simulink model "LQRAirrefuelingYingHu_full"  (R2013a)
settings: Solver=ode45  StartTime=0.0  StopTime=100  RelTol=1e-3
values from neighbouring files (symbols this model uses):
  A_full = [A_full(1:7,1:7),zeros(7,1),A_full(1:7,8:11) ... (first row only)    [LQR_Calc2_F16YingHu_lonAndLa.m]
  B_full = [zeros(1,4);B(1:6,1:4);zeros(1,4);B(7:10,1:4)]    [LQR_Calc2_F16YingHu_lonAndLa.m]
  C_xd_h_yd = [C_xd_h,zeros(2,5) ... (first row only)    [LQR_Calc2_F16YingHu_lonAndLa.m]
  Ki = zeros(4,3)    [F16NolinearModelRemoveWindControlData_low.m]    (also in F16_2003hiModelAutopilot.m; F16_2003hiModelAutopilot1.m; LQR_Calc2.m = -k(:,9:10); LQR_Calc2LowPrecision.m = -k(:,9:10))
  Kp = zeros(4,18)    [F16NolinearModelRemoveWindControlData_low.m]    (also in F16_2003hiModelAutopilot.m; F16_2003hiModelAutopilot1.m; F16_2003hiModelAutopilot1_steadySys.m; LQR_Calc2.m = k(:,1:8))
libraries: simulink x3
settings Model: Creator=Dai  LastModifiedBy=Dai

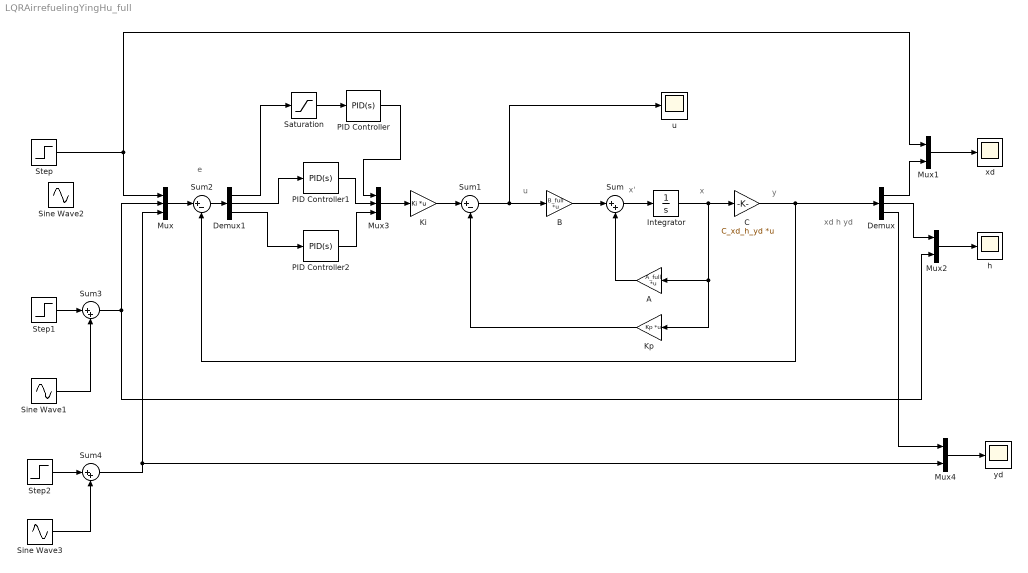
== system LQRAirrefuelingYingHu_full ==
  note: x
  note: x'
  note: y
  note: u
  note: xd
      | h
      | yd
  note: e
  A : Gain  Gain=A_full  Multiplication=Matrix(K*u) (u vector)
  B : Gain  Gain=B_full  Multiplication=Matrix(K*u) (u vector)
  C : Gain  Gain=C_xd_h_yd  Multiplication=Matrix(K*u) (u vector)
  Demux : Demux  Outputs=3
  Demux1 : Demux  Outputs=3
  Integrator : Integrator
  Ki : Gain  Gain=Ki  Multiplication=Matrix(K*u) (u vector)
  Kp : Gain  Gain=Kp  Multiplication=Matrix(K*u) (u vector)
  Mux : Mux  Inputs=3
  Mux1 : Mux  Inputs=2
  Mux2 : Mux  Inputs=2
  Mux3 : Mux  Inputs=3
  Mux4 : Mux  Inputs=2
  PID Controller : simulink/Continuous/PID Controller  Controller=PID  TimeDomain=Continuous-time  SampleTime=1  IntegratorMethod=Forward Euler  FilterMethod=Forward Euler  Form=Parallel  P=0  I=1.2  D=0  N=100  InitialConditionSource=internal  InitialConditionForIntegrator=0  InitialConditionForFilter=0  ExternalReset=none  LimitOutput=off  UpperSaturationLimit=inf  LowerSaturationLimit=-inf  LinearizeAsGain=on  AntiWindupMode=none  Kb=1  TrackingMode=off  Kt=1  PParamMin=[]  PParamMax=[]  IParamMin=[]  IParamMax=[]  DParamMin=[]  DParamMax=[]  NParamMin=[]  NParamMax=[]  KbParamMin=[]  KbParamMax=[]  KtParamMin=[]  KtParamMax=[]  POutMin=[]  POutMax=[]  IOutMin=[]  IOutMax=[]  DOutMin=[]  DOutMax=[]  NOutMin=[]  NOutMax=[]  KbOutMin=[]  KbOutMax=[]  KtOutMin=[]  KtOutMax=[]  IntegratorOutMin=[]  IntegratorOutMax=[]  FilterOutMin=[]  FilterOutMax=[]  SumOutMin=[]  SumOutMax=[]  SumI1OutMin=[]  SumI1OutMax=[]  SumI2OutMin=[]  SumI2OutMax=[]  SumI3OutMin=[]  SumI3OutMax=[]  SumDOutMin=[]  SumDOutMax=[]  SaturationOutMin=[]  SaturationOutMax=[]  IntegratorContinuousStateAttributes=''  IntegratorStateMustResolveToSignalObject=off  IntegratorRTWStateStorageClass=Auto  FilterContinuousStateAttributes=''  FilterStateMustResolveToSignalObject=off  FilterRTWStateStorageClass=Auto
  PID Controller1 : simulink/Continuous/PID Controller  Controller=PID  TimeDomain=Continuous-time  SampleTime=1  IntegratorMethod=Forward Euler  FilterMethod=Forward Euler  Form=Parallel  P=0  I=1.5  D=0  N=100  InitialConditionSource=internal  InitialConditionForIntegrator=0  InitialConditionForFilter=0  ExternalReset=none  LimitOutput=off  UpperSaturationLimit=inf  LowerSaturationLimit=-inf  LinearizeAsGain=on  AntiWindupMode=none  Kb=1  TrackingMode=off  Kt=1  PParamMin=[]  PParamMax=[]  IParamMin=[]  IParamMax=[]  DParamMin=[]  DParamMax=[]  NParamMin=[]  NParamMax=[]  KbParamMin=[]  KbParamMax=[]  KtParamMin=[]  KtParamMax=[]  POutMin=[]  POutMax=[]  IOutMin=[]  IOutMax=[]  DOutMin=[]  DOutMax=[]  NOutMin=[]  NOutMax=[]  KbOutMin=[]  KbOutMax=[]  KtOutMin=[]  KtOutMax=[]  IntegratorOutMin=[]  IntegratorOutMax=[]  FilterOutMin=[]  FilterOutMax=[]  SumOutMin=[]  SumOutMax=[]  SumI1OutMin=[]  SumI1OutMax=[]  SumI2OutMin=[]  SumI2OutMax=[]  SumI3OutMin=[]  SumI3OutMax=[]  SumDOutMin=[]  SumDOutMax=[]  SaturationOutMin=[]  SaturationOutMax=[]  IntegratorContinuousStateAttributes=''  IntegratorStateMustResolveToSignalObject=off  IntegratorRTWStateStorageClass=Auto  FilterContinuousStateAttributes=''  FilterStateMustResolveToSignalObject=off  FilterRTWStateStorageClass=Auto
  PID Controller2 : simulink/Continuous/PID Controller  Controller=PID  TimeDomain=Continuous-time  SampleTime=1  IntegratorMethod=Forward Euler  FilterMethod=Forward Euler  Form=Parallel  P=0  I=1  D=0  N=100  InitialConditionSource=internal  InitialConditionForIntegrator=0  InitialConditionForFilter=0  ExternalReset=none  LimitOutput=off  UpperSaturationLimit=inf  LowerSaturationLimit=-inf  LinearizeAsGain=on  AntiWindupMode=none  Kb=1  TrackingMode=off  Kt=1  PParamMin=[]  PParamMax=[]  IParamMin=[]  IParamMax=[]  DParamMin=[]  DParamMax=[]  NParamMin=[]  NParamMax=[]  KbParamMin=[]  KbParamMax=[]  KtParamMin=[]  KtParamMax=[]  POutMin=[]  POutMax=[]  IOutMin=[]  IOutMax=[]  DOutMin=[]  DOutMax=[]  NOutMin=[]  NOutMax=[]  KbOutMin=[]  KbOutMax=[]  KtOutMin=[]  KtOutMax=[]  IntegratorOutMin=[]  IntegratorOutMax=[]  FilterOutMin=[]  FilterOutMax=[]  SumOutMin=[]  SumOutMax=[]  SumI1OutMin=[]  SumI1OutMax=[]  SumI2OutMin=[]  SumI2OutMax=[]  SumI3OutMin=[]  SumI3OutMax=[]  SumDOutMin=[]  SumDOutMax=[]  SaturationOutMin=[]  SaturationOutMax=[]  IntegratorContinuousStateAttributes=''  IntegratorStateMustResolveToSignalObject=off  IntegratorRTWStateStorageClass=Auto  FilterContinuousStateAttributes=''  FilterStateMustResolveToSignalObject=off  FilterRTWStateStorageClass=Auto
  Saturation : Saturate
  Sine Wave1 : Sin  Amplitude=0.2  Frequency=0.05  SampleTime=0
  Sine Wave2 : Sin  Amplitude=5  Frequency=0.05  SampleTime=0
  Sine Wave3 : Sin  Amplitude=0.2  Frequency=0.05  SampleTime=0
  Step : Step  After=5  SampleTime=0
  Step1 : Step  Time=0  After=5  SampleTime=0
  Step2 : Step  Time=0  After=5  SampleTime=0
  Sum : Sum  Inputs=|++
  Sum1 : Sum  Inputs=|+-
  Sum2 : Sum  Inputs=|+-
  Sum3 : Sum  Inputs=|++
  Sum4 : Sum  Inputs=|++
  h : Scope
  u : Scope
      settings: SaveName=ScopeData2
  xd : Scope
  yd : Scope
      settings: SaveName=ScopeData3
  wires:
  Integrator/1 -> C/1, A/1, Kp/1
  B/1 -> Sum/1
  Sum/1 -> Integrator/1
  A/1 -> Sum/2
  Ki/1 -> Sum1/1
  C/1 -> Demux/1, Sum2/2
  Mux/1 -> Sum2/1
  Step/1 -> Mux/1, Mux1/1
  Demux/1 -> Mux1/2
  Mux1/1 -> xd/1
  Sum3/1 -> Mux2/2, Mux/2
  Mux2/1 -> h/1
  Demux/2 -> Mux2/1
  Kp/1 -> Sum1/2
  Sum2/1 -> Demux1/1
  Mux3/1 -> Ki/1
  Sum1/1 -> u/1, B/1
  Demux1/1 -> Saturation/1
  Demux1/2 -> PID Controller1/1
  PID Controller/1 -> Mux3/1
  PID Controller1/1 -> Mux3/2
  Saturation/1 -> PID Controller/1
  Step1/1 -> Sum3/1
  Sine Wave1/1 -> Sum3/2
  Demux1/3 -> PID Controller2/1
  PID Controller2/1 -> Mux3/3
  Sum4/1 -> Mux4/2, Mux/3
  Mux4/1 -> yd/1
  Demux/3 -> Mux4/1
  Step2/1 -> Sum4/1
  Sine Wave3/1 -> Sum4/2
